simulink model "experiment_setup_R2019b"  (R2020a)
settings: Solver=FixedStepAuto  StartTime=0.0  StopTime=inf  FixedStep=1  RelTol=1e-3
libraries: modbusMatLib x8, simulink x4, realtime_pacer_lib x2
settings Model: Creator=pppc  LastModifiedBy=Casper and Adis
settings DebuggingCC: InheritedTsInSrcMsg=none
settings SFSimCC: CustomCodeUndefinedFunction=UseInterfaceOnly

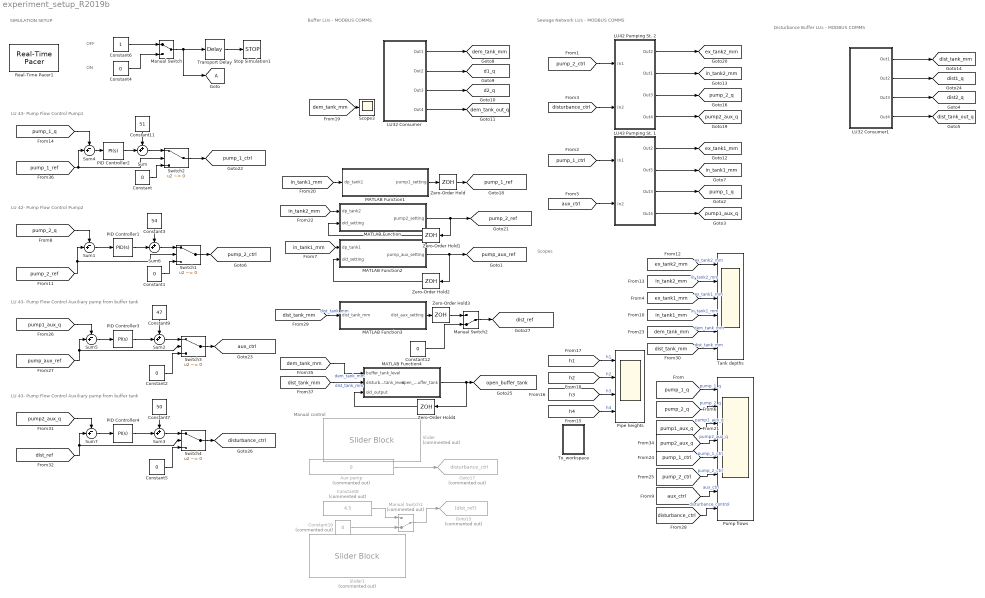
== system experiment_setup_R2019b ==
  note: Buffer LUs - MODBUS COMMS
  note: LU 43- Pump Flow Control Auxiliary pump from buffer tank
  note: Manual control
  note: OFF
  note: SIMULATION SETUP
  note: Sewage Network LUs - MODBUS COMMS
  note: LU 43- Pump Flow Control Pump1
  note: LU 42- Pump Flow Control Pump2
  note: ON
  note: Scopes
  note: Disturbance Buffer LUs - MODBUS COMMS
  note: LU 43- Pump Flow Control Auxiliary pump from buffer tank
  Aux pump : Constant  Commented=on  Value=0
  Constant{,1..2,4..5,12} (6 alike) : Constant  Value=0
  Constant10 : Constant  Commented=on  Value=0
  Constant11 : Constant  Value=51
  Constant3 : Constant  Value=54
  Constant6 : Constant
  Constant7 : Constant  Value=50
  Constant8 : Constant  Commented=on  Value=4.5
  Constant9 : Constant  Value=47
  Goto15 : Goto  Commented=on  GotoTag=dist_ref
  Goto17 : Goto  Commented=on  GotoTag=disturbance_ctrl  TagVisibility=global
  LU32 Consumer : Subsystem
  LU32 Consumer1 : Subsystem
  LU42 Pumping St. 2 : Subsystem
  LU43 Pumping St. 1 : Subsystem
  MATLAB Function : MATLAB Function  TreatAsAtomicUnit=on
  MATLAB Function1 : MATLAB Function  TreatAsAtomicUnit=on
  MATLAB Function2 : MATLAB Function  TreatAsAtomicUnit=on
  MATLAB Function3 : MATLAB Function  TreatAsAtomicUnit=on
  MATLAB Function4 : MATLAB Function  TreatAsAtomicUnit=on
  Manual Switch : ManualSwitch
  Manual Switch1 : ManualSwitch  Commented=on  CurrentSetting=0
  Manual Switch2 : ManualSwitch  CurrentSetting=0
  PID Controller1 : simulink/Continuous/PID Controller  Controller=PID  Form=Parallel  TimeDomain=Continuous-time  UseExternalTs=off  SampleTime=1  IntegratorMethod=Forward Euler  FilterMethod=Forward Euler  ControllerParametersSource=internal  P=0.145  I=0.61  D=0  UseFilter=on  N=100  TunerSelectOption=Transfer Function Based (PID Tuner App)  InitialConditionSource=internal  InitialConditionForIntegrator=0  InitialConditionForFilter=0  DifferentiatorICPrevScaledInput=0  ExternalReset=none  TrackingMode=off  Kt=1  LimitOutput=on  UpperSaturationLimit=46  LowerSaturationLimit=0  LinearizeAsGain=off  AntiWindupMode=clamping  Kb=1  POutMin=[]  POutMax=[]  IOutMin=[]  IOutMax=[]  DOutMin=[]  DOutMax=[]  NOutMin=[]  NOutMax=[]  SumOutMin=[]  SumOutMax=[]  SaturationOutMin=[]  SaturationOutMax=[]  PParamMin=[]  PParamMax=[]  IParamMin=[]  IParamMax=[]  DParamMin=[]  DParamMax=[]  NParamMin=[]  NParamMax=[]  KbParamMin=[]  KbParamMax=[]  KtParamMin=[]  KtParamMax=[]  KbOutMin=[]  KbOutMax=[]  KtOutMin=[]  KtOutMax=[]  IntegratorOutMin=[]  IntegratorOutMax=[]  FilterOutMin=[]  FilterOutMax=[]  SumI1OutMin=[]  SumI1OutMax=[]  SumI2OutMin=[]  SumI2OutMax=[]  SumI3OutMin=[]  SumI3OutMax=[]  SumI4OutMin=[]  SumI4OutMax=[]  SumDOutMin=[]  SumDOutMax=[]  DifferentiatorOutMin=[]  DifferentiatorOutMax=[]  FilterDiffOutCoefMin=[]  FilterDiffOutCoefMax=[]  ReciprocalOutMin=[]  ReciprocalOutMax=[]  SumDenOutMin=[]  SumDenOutMax=[]  SumNumOutMin=[]  SumNumOutMax=[]  DivideOutMin=[]  DivideOutMax=[]  UdiffTsProdOutMin=[]  UdiffTsProdOutMax=[]  NTsProdOutMin=[]  NTsProdOutMax=[]  UintegralTsProdOutMin=[]  UintegralTsProdOutMax=[]  UngainTsProdOutMin=[]  UngainTsProdOutMax=[]  IntegratorContinuousStateAttributes=''  IntegratorStateMustResolveToSignalObject=off  IntegratorRTWStateStorageClass=Auto  FilterContinuousStateAttributes=''  FilterStateMustResolveToSignalObject=off  FilterRTWStateStorageClass=Auto  ParallelPVariant=InternalParameters  IdealPVariant=Disabled  IVariant=InternalParameters  DVariant=InternalParameters  IntegratorVariant=Continuous  SatVariant=Enabled  AWVariant=ContClampingParallel  PCopyVariant=Disabled  TRVariant=Disabled  FdbkBlocksVariant=Forward  IdealPFdbkVariant=Disabled  SatFdbkVariant=Disabled  DerivativeFilterVariant=ContFilter  NVariant=InternalParameters  NCopyVariant=Disabled  FilterICVariant=InternalICsFilter  IntegratorICVariant=InternalICs  ExternalResetVariant=Disabled  TRSumVariant=Passthrough  SumFdbkVariant=Disabled  SumVariant=Sum_PID  TsampFilterVariant=InternalTs  TsampNgainVariant=Passthrough  TsampIntegralVariant=Passthrough
  PID Controller2 : simulink/Continuous/PID Controller  Controller=PI  Form=Parallel  TimeDomain=Continuous-time  UseExternalTs=off  SampleTime=1  IntegratorMethod=Forward Euler  FilterMethod=Forward Euler  ControllerParametersSource=internal  P=0.1  I=0.3  D=0  UseFilter=on  N=100  TunerSelectOption=Transfer Function Based (PID Tuner App)  InitialConditionSource=internal  InitialConditionForIntegrator=0  InitialConditionForFilter=0  DifferentiatorICPrevScaledInput=0  ExternalReset=none  TrackingMode=off  Kt=1  LimitOutput=on  UpperSaturationLimit=49  LowerSaturationLimit=0  LinearizeAsGain=off  AntiWindupMode=clamping  Kb=1  POutMin=[]  POutMax=[]  IOutMin=[]  IOutMax=[]  DOutMin=[]  DOutMax=[]  NOutMin=[]  NOutMax=[]  SumOutMin=[]  SumOutMax=[]  SaturationOutMin=[]  SaturationOutMax=[]  PParamMin=[]  PParamMax=[]  IParamMin=[]  IParamMax=[]  DParamMin=[]  DParamMax=[]  NParamMin=[]  NParamMax=[]  KbParamMin=[]  KbParamMax=[]  KtParamMin=[]  KtParamMax=[]  KbOutMin=[]  KbOutMax=[]  KtOutMin=[]  KtOutMax=[]  IntegratorOutMin=[]  IntegratorOutMax=[]  FilterOutMin=[]  FilterOutMax=[]  SumI1OutMin=[]  SumI1OutMax=[]  SumI2OutMin=[]  SumI2OutMax=[]  SumI3OutMin=[]  SumI3OutMax=[]  SumI4OutMin=[]  SumI4OutMax=[]  SumDOutMin=[]  SumDOutMax=[]  DifferentiatorOutMin=[]  DifferentiatorOutMax=[]  FilterDiffOutCoefMin=[]  FilterDiffOutCoefMax=[]  ReciprocalOutMin=[]  ReciprocalOutMax=[]  SumDenOutMin=[]  SumDenOutMax=[]  SumNumOutMin=[]  SumNumOutMax=[]  DivideOutMin=[]  DivideOutMax=[]  UdiffTsProdOutMin=[]  UdiffTsProdOutMax=[]  NTsProdOutMin=[]  NTsProdOutMax=[]  UintegralTsProdOutMin=[]  UintegralTsProdOutMax=[]  UngainTsProdOutMin=[]  UngainTsProdOutMax=[]  IntegratorContinuousStateAttributes=''  IntegratorStateMustResolveToSignalObject=off  IntegratorRTWStateStorageClass=Auto  FilterContinuousStateAttributes=''  FilterStateMustResolveToSignalObject=off  FilterRTWStateStorageClass=Auto  ParallelPVariant=InternalParameters  IdealPVariant=Disabled  IVariant=InternalParameters  DVariant=Disabled  IntegratorVariant=Continuous  SatVariant=Enabled  AWVariant=ContClampingParallel  PCopyVariant=Disabled  TRVariant=Disabled  FdbkBlocksVariant=Forward  IdealPFdbkVariant=Disabled  SatFdbkVariant=Disabled  DerivativeFilterVariant=Disabled  NVariant=Disabled  NCopyVariant=Disabled_SignalSpec  FilterICVariant=Disabled  IntegratorICVariant=InternalICs  ExternalResetVariant=Disabled  TRSumVariant=Passthrough  SumFdbkVariant=Disabled  SumVariant=Sum_PI  TsampFilterVariant=InternalTs  TsampNgainVariant=Passthrough  TsampIntegralVariant=Passthrough
  PID Controller3 : simulink/Continuous/PID Controller  Controller=PI  Form=Parallel  TimeDomain=Continuous-time  UseExternalTs=off  SampleTime=1  IntegratorMethod=Forward Euler  FilterMethod=Forward Euler  ControllerParametersSource=internal  P=0.15  I=0.45  D=0  UseFilter=on  N=100  TunerSelectOption=Transfer Function Based (PID Tuner App)  InitialConditionSource=internal  InitialConditionForIntegrator=0  InitialConditionForFilter=0  DifferentiatorICPrevScaledInput=0  ExternalReset=none  TrackingMode=off  Kt=1  LimitOutput=on  UpperSaturationLimit=53  LowerSaturationLimit=0  LinearizeAsGain=off  AntiWindupMode=clamping  Kb=1  POutMin=[]  POutMax=[]  IOutMin=[]  IOutMax=[]  DOutMin=[]  DOutMax=[]  NOutMin=[]  NOutMax=[]  SumOutMin=[]  SumOutMax=[]  SaturationOutMin=[]  SaturationOutMax=[]  PParamMin=[]  PParamMax=[]  IParamMin=[]  IParamMax=[]  DParamMin=[]  DParamMax=[]  NParamMin=[]  NParamMax=[]  KbParamMin=[]  KbParamMax=[]  KtParamMin=[]  KtParamMax=[]  KbOutMin=[]  KbOutMax=[]  KtOutMin=[]  KtOutMax=[]  IntegratorOutMin=[]  IntegratorOutMax=[]  FilterOutMin=[]  FilterOutMax=[]  SumI1OutMin=[]  SumI1OutMax=[]  SumI2OutMin=[]  SumI2OutMax=[]  SumI3OutMin=[]  SumI3OutMax=[]  SumI4OutMin=[]  SumI4OutMax=[]  SumDOutMin=[]  SumDOutMax=[]  DifferentiatorOutMin=[]  DifferentiatorOutMax=[]  FilterDiffOutCoefMin=[]  FilterDiffOutCoefMax=[]  ReciprocalOutMin=[]  ReciprocalOutMax=[]  SumDenOutMin=[]  SumDenOutMax=[]  SumNumOutMin=[]  SumNumOutMax=[]  DivideOutMin=[]  DivideOutMax=[]  UdiffTsProdOutMin=[]  UdiffTsProdOutMax=[]  NTsProdOutMin=[]  NTsProdOutMax=[]  UintegralTsProdOutMin=[]  UintegralTsProdOutMax=[]  UngainTsProdOutMin=[]  UngainTsProdOutMax=[]  IntegratorContinuousStateAttributes=''  IntegratorStateMustResolveToSignalObject=off  IntegratorRTWStateStorageClass=Auto  FilterContinuousStateAttributes=''  FilterStateMustResolveToSignalObject=off  FilterRTWStateStorageClass=Auto  ParallelPVariant=InternalParameters  IdealPVariant=Disabled  IVariant=InternalParameters  DVariant=Disabled  IntegratorVariant=Continuous  SatVariant=Enabled  AWVariant=ContClampingParallel  PCopyVariant=Disabled  TRVariant=Disabled  FdbkBlocksVariant=Forward  IdealPFdbkVariant=Disabled  SatFdbkVariant=Disabled  DerivativeFilterVariant=Disabled  NVariant=Disabled  NCopyVariant=Disabled_SignalSpec  FilterICVariant=Disabled  IntegratorICVariant=InternalICs  ExternalResetVariant=Disabled  TRSumVariant=Passthrough  SumFdbkVariant=Disabled  SumVariant=Sum_PI  TsampFilterVariant=InternalTs  TsampNgainVariant=Passthrough  TsampIntegralVariant=Passthrough
  PID Controller4 : simulink/Continuous/PID Controller  Controller=PI  Form=Parallel  TimeDomain=Continuous-time  UseExternalTs=off  SampleTime=1  IntegratorMethod=Forward Euler  FilterMethod=Forward Euler  ControllerParametersSource=internal  P=0.1  I=0.4  D=0  UseFilter=on  N=100  TunerSelectOption=Transfer Function Based (PID Tuner App)  InitialConditionSource=internal  InitialConditionForIntegrator=0  InitialConditionForFilter=0  DifferentiatorICPrevScaledInput=0  ExternalReset=none  TrackingMode=off  Kt=1  LimitOutput=on  UpperSaturationLimit=53  LowerSaturationLimit=0  LinearizeAsGain=off  AntiWindupMode=clamping  Kb=1  POutMin=[]  POutMax=[]  IOutMin=[]  IOutMax=[]  DOutMin=[]  DOutMax=[]  NOutMin=[]  NOutMax=[]  SumOutMin=[]  SumOutMax=[]  SaturationOutMin=[]  SaturationOutMax=[]  PParamMin=[]  PParamMax=[]  IParamMin=[]  IParamMax=[]  DParamMin=[]  DParamMax=[]  NParamMin=[]  NParamMax=[]  KbParamMin=[]  KbParamMax=[]  KtParamMin=[]  KtParamMax=[]  KbOutMin=[]  KbOutMax=[]  KtOutMin=[]  KtOutMax=[]  IntegratorOutMin=[]  IntegratorOutMax=[]  FilterOutMin=[]  FilterOutMax=[]  SumI1OutMin=[]  SumI1OutMax=[]  SumI2OutMin=[]  SumI2OutMax=[]  SumI3OutMin=[]  SumI3OutMax=[]  SumI4OutMin=[]  SumI4OutMax=[]  SumDOutMin=[]  SumDOutMax=[]  DifferentiatorOutMin=[]  DifferentiatorOutMax=[]  FilterDiffOutCoefMin=[]  FilterDiffOutCoefMax=[]  ReciprocalOutMin=[]  ReciprocalOutMax=[]  SumDenOutMin=[]  SumDenOutMax=[]  SumNumOutMin=[]  SumNumOutMax=[]  DivideOutMin=[]  DivideOutMax=[]  UdiffTsProdOutMin=[]  UdiffTsProdOutMax=[]  NTsProdOutMin=[]  NTsProdOutMax=[]  UintegralTsProdOutMin=[]  UintegralTsProdOutMax=[]  UngainTsProdOutMin=[]  UngainTsProdOutMax=[]  IntegratorContinuousStateAttributes=''  IntegratorStateMustResolveToSignalObject=off  IntegratorRTWStateStorageClass=Auto  FilterContinuousStateAttributes=''  FilterStateMustResolveToSignalObject=off  FilterRTWStateStorageClass=Auto  ParallelPVariant=InternalParameters  IdealPVariant=Disabled  IVariant=InternalParameters  DVariant=Disabled  IntegratorVariant=Continuous  SatVariant=Enabled  AWVariant=ContClampingParallel  PCopyVariant=Disabled  TRVariant=Disabled  FdbkBlocksVariant=Forward  IdealPFdbkVariant=Disabled  SatFdbkVariant=Disabled  DerivativeFilterVariant=Disabled  NVariant=Disabled  NCopyVariant=Disabled_SignalSpec  FilterICVariant=Disabled  IntegratorICVariant=InternalICs  ExternalResetVariant=Disabled  TRSumVariant=Passthrough  SumFdbkVariant=Disabled  SumVariant=Sum_PI  TsampFilterVariant=InternalTs  TsampNgainVariant=Passthrough  TsampIntegralVariant=Passthrough
  Pipe heights : Scope  NumInputPorts=4
  Pump flows : Scope  NumInputPorts=8
  Real-Time Pacer1 : realtime_pacer_lib/Real-Time Pacer  simTimePerRealTime=2
  Scope3 : Scope
  Slider : SliderBlock  Commented=on
  Slider1 : SliderBlock  Commented=on  ScaleMax=9.5
  Stop Simulation1 : Stop
  Sum{,2..3,6} (4 alike) : Sum  Inputs=++|
  Sum{1,4..5,7} (4 alike) : Sum  Inputs=-+|
  Switch{1..4} (4 alike) : Switch  Criteria=u2 ~= 0
  Tank depths : Scope  NumInputPorts=6
  To_workspace : Subsystem
  Transport Delay : TransportDelay  DelayTime=2
  Zero-Order Hold : ZeroOrderHold  SampleTime=60
  Zero-Order Hold1 : ZeroOrderHold  SampleTime=2
  Zero-Order Hold2 : ZeroOrderHold  SampleTime=2
  Zero-Order Hold3 : ZeroOrderHold  SampleTime=30
  Zero-Order Hold4 : ZeroOrderHold  SampleTime=2
  tag scope: A=global, aux_ctrl=global, d1_q=global, d2_q=global, dem_tank_mm=global, dem_tank_out_q=global, dist1_q=global, dist2_q=global, dist_ref=global, dist_tank_mm=global, dist_tank_out_q=global, disturbance_ctrl=global, ex_tank1_mm=global, ex_tank2_mm=global, in_tank1_mm=global, in_tank2_mm=global, open_buffer_tank=global, pump1_aux_q=global, pump2_aux_q=global, pump_1_ctrl=global, pump_1_q=global, pump_1_ref=global, pump_2_ctrl=global, pump_2_q=global, pump_2_ref=global, pump_aux_ref=global
  wires:
  [pump_1_q] -> Sum4/1
  [pump_aux_ref] -> Sum5/2, Switch3/2
  [disturbance_ctrl] -> LU42 Pumping St. 2/2(In2)
  [pump_2_ref] -> Switch1/2, Sum1/2
  [in_tank2_mm] -> Tank depths/2  "in_tank2_mm"
  [dem_tank_mm] -> Scope3/1
  MATLAB Function/1(pump2_setting) -> Zero-Order Hold1/1, [pump_2_ref]
  [pump_2_q] -> Pump flows/2  "pump_2_q"
  Switch1/1 -> [pump_2_ctrl]
  Sum6/1 -> Switch1/1
  PID Controller2/1 -> Sum/2
  PID Controller1/1 -> Sum6/2
  Switch3/1 -> [aux_ctrl]
  [pump_2_q] -> Sum1/1
  Sum2/1 -> Switch3/1
  LU42 Pumping St. 2/3(Out3) -> [pump_2_q]
  Zero-Order Hold/1 -> [pump_1_ref]
  Constant9/1 -> Sum2/1
  LU32 Consumer/4(Out4) -> [dem_tank_out_q]
  Constant2/1 -> Switch3/3
  PID Controller3/1 -> Sum2/2
  [h4] -> Pipe heights/4  "h4"
  Constant11/1 -> Sum/1
  [pump_1_ref] -> Sum4/2, Switch2/2
  [pump_1_ctrl] -> LU43 Pumping St. 1/1(In1)
  Constant3/1 -> Sum6/1
  LU43 Pumping St. 1/2(Out5) -> [in_tank1_mm]
  Sum/1 -> Switch2/1
  Transport Delay/1 -> Stop Simulation1/1
  Constant6/1 -> Manual Switch/1
  Constant/1 -> Switch2/3
  LU43 Pumping St. 1/1(Out2) -> [ex_tank1_mm]
  [in_tank1_mm] -> Tank depths/4  "in_tank1_mm"
  Aux pump/1 -> Goto17/1
  Constant4/1 -> Manual Switch/2
  [ex_tank1_mm] -> Tank depths/3  "ex_tank1_mm"
  [pump1_aux_q] -> Sum5/1
  [dem_tank_mm] -> Tank depths/5  "dem_tank_mm"
  Sum5/1 -> PID Controller3/1
  Manual Switch/1 -> [A], Transport Delay/1
  [pump_2_ctrl] -> LU42 Pumping St. 2/1(In1)
  LU42 Pumping St. 2/4(Out4) -> [pump2_aux_q]
  LU32 Consumer/3(Out3) -> [d2_q]
  LU32 Consumer/1(Out1) -> [dem_tank_mm]
  LU42 Pumping St. 2/1(Out2) -> [ex_tank2_mm]
  [in_tank1_mm] -> MATLAB Function1/1(dp_tank1)
  [in_tank2_mm] -> MATLAB Function/1(dp_tank2)
  Sum1/1 -> PID Controller1/1
  [ex_tank2_mm] -> Tank depths/1  "ex_tank2_mm"
  Switch2/1 -> [pump_1_ctrl]
  [h2] -> Pipe heights/2  "h2"
  [h3] -> Pipe heights/3  "h3"
  LU43 Pumping St. 1/3(Out3) -> [pump_1_q]
  Sum4/1 -> PID Controller2/1
  LU43 Pumping St. 1/4(Out4) -> [pump1_aux_q]
  [aux_ctrl] -> LU43 Pumping St. 1/2(In2)
  LU42 Pumping St. 2/2(Out1) -> [in_tank2_mm]
  LU32 Consumer/2(Out2) -> [d1_q]
  MATLAB Function1/1(pump1_setting) -> Zero-Order Hold/1
  Constant1/1 -> Switch1/3
  [in_tank1_mm] -> MATLAB Function2/1(dp_tank1)
  MATLAB Function2/1(pump_aux_setting) -> Zero-Order Hold2/1, [pump_aux_ref]
  Zero-Order Hold1/1 -> MATLAB Function/2(old_setting)
  Zero-Order Hold2/1 -> MATLAB Function2/2(old_setting)
  [pump1_aux_q] -> Pump flows/3  "pump1_aux_q"
  [pump_1_q] -> Pump flows/1  "pump_1_q"
  LU32 Consumer1/2(Out2) -> [dist1_q]
  LU32 Consumer1/3(Out3) -> [dist2_q]
  LU32 Consumer1/4(Out4) -> [dist_tank_out_q]
  LU32 Consumer1/1(Out1) -> [dist_tank_mm]
  [dist_tank_mm] -> Tank depths/6  "dist_tank_mm"
  [pump2_aux_q] -> Sum7/1
  Constant7/1 -> Sum3/1
  Switch4/1 -> [disturbance_ctrl]
  PID Controller4/1 -> Sum3/2
  [dist_ref] -> Sum7/2, Switch4/2
  Sum3/1 -> Switch4/1
  Sum7/1 -> PID Controller4/1
  Constant5/1 -> Switch4/3
  [pump_1_ctrl] -> Pump flows/5  "pump_1_ctrl"
  [pump_2_ctrl] -> Pump flows/6  "pump_2_ctrl"
  [aux_ctrl] -> Pump flows/7  "aux_ctrl"
  [disturbance_ctrl] -> Pump flows/8  "disturbance_control"
  [pump2_aux_q] -> Pump flows/4  "pump2_aux_q"
  [dem_tank_mm] -> MATLAB Function4/1(buffer_tank_level)  "dem_tank_mm"
  [dist_tank_mm] -> MATLAB Function4/2(disturbance_tank_level)  "dist_tank_mm"
  MATLAB Function4/1(open_buffer_tank) -> Zero-Order Hold4/1, [open_buffer_tank]
  Zero-Order Hold4/1 -> MATLAB Function4/3(old_output)
  [h1] -> Pipe heights/1  "h1"
  Constant8/1 -> Manual Switch1/1
  Constant10/1 -> Manual Switch1/2
  Manual Switch1/1 -> Goto15/1
  [dist_tank_mm] -> MATLAB Function3/1(dist_tank_mm)  "dist_tank_mm"
  MATLAB Function3/1(dist_aux_setting) -> Zero-Order Hold3/1
  Zero-Order Hold3/1 -> Manual Switch2/1
  Manual Switch2/1 -> [dist_ref]
  Constant12/1 -> Manual Switch2/2

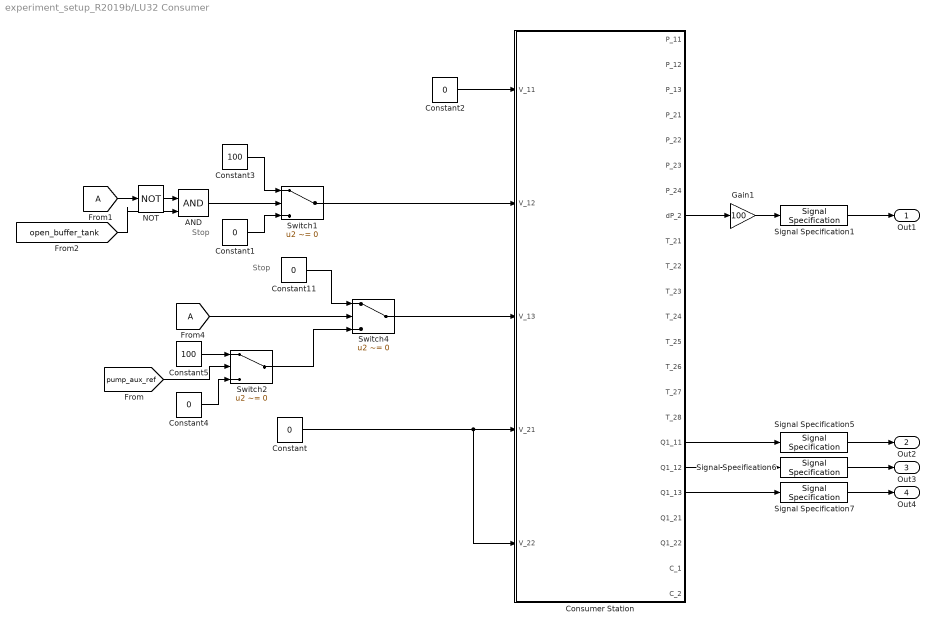
== system experiment_setup_R2019b/LU32 Consumer ==
  note: Stop
  note: Stop
  AND : Logic  IconShape=distinctive  AllPortsSameDT=off  OutDataTypeStr=boolean
  Constant{,1..2,4,11} (5 alike) : Constant  Value=0
  Constant3 : Constant  Value=100
  Constant5 : Constant  Value=100
  Consumer Station : Subsystem
  Gain1 : Gain  Gain=100
  NOT : Logic  Operator=NOT  IconShape=distinctive  AllPortsSameDT=off  OutDataTypeStr=boolean
  Signal Specification1 : SignalSpecification  Unit=mm
  Signal Specification5 : SignalSpecification  Unit=l/min
  Signal Specification6 : SignalSpecification  Unit=l/min
  Signal Specification7 : SignalSpecification  Unit=l/min
  Switch1 : Switch  Criteria=u2 ~= 0
  Switch2 : Switch  Criteria=u2 ~= 0
  Switch4 : Switch  Criteria=u2 ~= 0
  Out1 : Outport  VectorParamsAs1DForOutWhenUnconnected=off
  Out2 : Outport  Port=2  VectorParamsAs1DForOutWhenUnconnected=off
  Out3 : Outport  Port=3  VectorParamsAs1DForOutWhenUnconnected=off
  Out4 : Outport  Port=4  VectorParamsAs1DForOutWhenUnconnected=off
  wires:
  Consumer Station/8(dP_2) -> Gain1/1
  Switch4/1 -> Consumer Station/3(V_13)
  Consumer Station/19(Q1_13) -> Signal Specification7/1
  Consumer Station/17(Q1_11) -> Signal Specification5/1
  Consumer Station/18(Q1_12) -> Signal Specification6/1
  Gain1/1 -> Signal Specification1/1
  [A] -> Switch4/2
  Signal Specification7/1 -> Out4/1
  Constant11/1 -> Switch4/1
  Signal Specification5/1 -> Out2/1
  Constant/1 -> Consumer Station/5(V_22), Consumer Station/4(V_21)
  Signal Specification6/1 -> Out3/1
  Signal Specification1/1 -> Out1/1
  Switch1/1 -> Consumer Station/2(V_12)
  Constant2/1 -> Consumer Station/1(V_11)
  [pump_aux_ref] -> Switch2/2
  Switch2/1 -> Switch4/3
  Constant5/1 -> Switch2/1
  Constant4/1 -> Switch2/3
  [A] -> NOT/1
  NOT/1 -> AND/1
  AND/1 -> Switch1/2
  Constant1/1 -> Switch1/3
  Constant3/1 -> Switch1/1
  [open_buffer_tank] -> AND/2

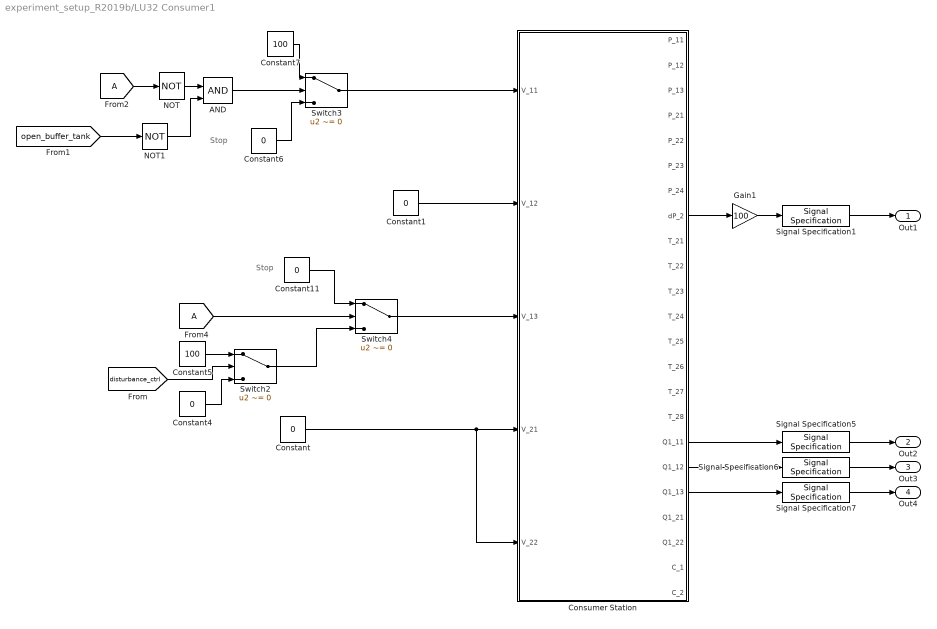
== system experiment_setup_R2019b/LU32 Consumer1 ==
  note: Stop
  note: Stop
  AND : Logic  IconShape=distinctive  AllPortsSameDT=off  OutDataTypeStr=boolean
  Constant{,1,4,6,11} (5 alike) : Constant  Value=0
  Constant5 : Constant  Value=100
  Constant7 : Constant  Value=100
  Consumer Station : Subsystem
  Gain1 : Gain  Gain=100
  NOT : Logic  Operator=NOT  IconShape=distinctive  AllPortsSameDT=off  OutDataTypeStr=boolean
  NOT1 : Logic  Operator=NOT  IconShape=distinctive  AllPortsSameDT=off  OutDataTypeStr=boolean
  Signal Specification1 : SignalSpecification  Unit=mm
  Signal Specification5 : SignalSpecification  Unit=l/min
  Signal Specification6 : SignalSpecification  Unit=l/min
  Signal Specification7 : SignalSpecification  Unit=l/min
  Switch2 : Switch  Criteria=u2 ~= 0
  Switch3 : Switch  Criteria=u2 ~= 0
  Switch4 : Switch  Criteria=u2 ~= 0
  Out1 : Outport  VectorParamsAs1DForOutWhenUnconnected=off
  Out2 : Outport  Port=2  VectorParamsAs1DForOutWhenUnconnected=off
  Out3 : Outport  Port=3  VectorParamsAs1DForOutWhenUnconnected=off
  Out4 : Outport  Port=4  VectorParamsAs1DForOutWhenUnconnected=off
  wires:
  Consumer Station/8(dP_2) -> Gain1/1
  Switch4/1 -> Consumer Station/3(V_13)
  Consumer Station/19(Q1_13) -> Signal Specification7/1
  Consumer Station/17(Q1_11) -> Signal Specification5/1
  Consumer Station/18(Q1_12) -> Signal Specification6/1
  Gain1/1 -> Signal Specification1/1
  [A] -> Switch4/2
  Signal Specification7/1 -> Out4/1
  Constant11/1 -> Switch4/1
  Signal Specification5/1 -> Out2/1
  Constant/1 -> Consumer Station/5(V_22), Consumer Station/4(V_21)
  Signal Specification6/1 -> Out3/1
  Signal Specification1/1 -> Out1/1
  Switch3/1 -> Consumer Station/1(V_11)
  [disturbance_ctrl] -> Switch2/2
  Switch2/1 -> Switch4/3
  Constant5/1 -> Switch2/1
  Constant4/1 -> Switch2/3
  Constant1/1 -> Consumer Station/2(V_12)
  [A] -> NOT/1
  Constant6/1 -> Switch3/3
  Constant7/1 -> Switch3/1
  AND/1 -> Switch3/2
  NOT/1 -> AND/1
  [open_buffer_tank] -> NOT1/1
  NOT1/1 -> AND/2

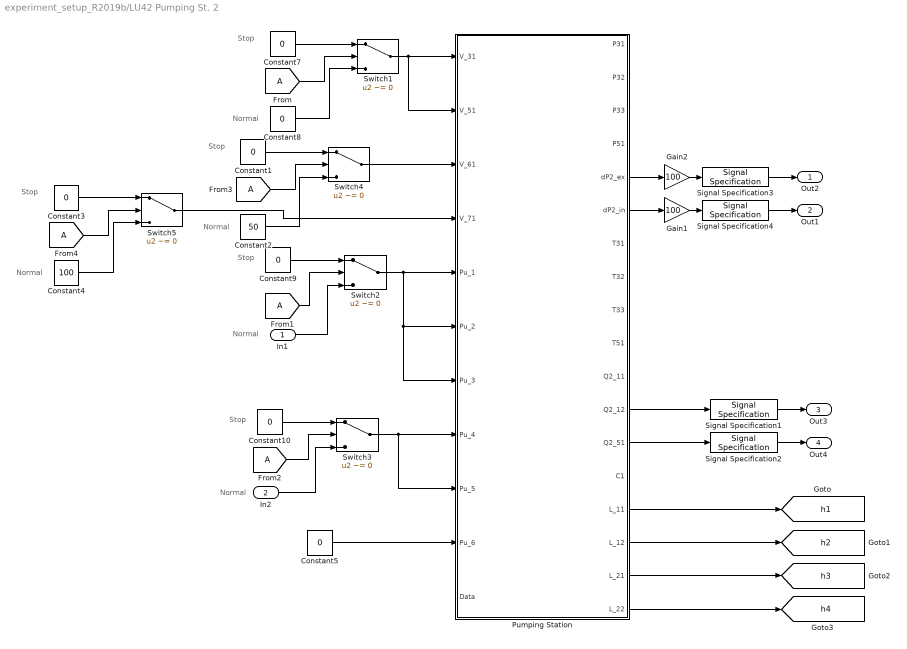
== system experiment_setup_R2019b/LU42 Pumping St. 2 ==
  note: Stop
  note: Stop
  note: Normal
  note: Stop
  note: Normal
  note: Normal
  note: Stop
  note: Normal
  note: Normal
  note: Stop
  In1 : Inport
  In2 : Inport  Port=2
  Constant{1,3,5,7..10} (7 alike) : Constant  Value=0
  Constant2 : Constant  Value=50
  Constant4 : Constant  Value=100
  Gain1 : Gain  Gain=100
  Gain2 : Gain  Gain=100
  Pumping Station : Subsystem
  Signal Specification1 : SignalSpecification  Unit=l/min
  Signal Specification2 : SignalSpecification  Unit=l/min
  Signal Specification3 : SignalSpecification  Unit=mm
  Signal Specification4 : SignalSpecification  Unit=mm
  Switch{1..5} (5 alike) : Switch  Criteria=u2 ~= 0
  Out2 : Outport  VectorParamsAs1DForOutWhenUnconnected=off
  Out1 : Outport  Port=2  VectorParamsAs1DForOutWhenUnconnected=off
  Out3 : Outport  Port=3  VectorParamsAs1DForOutWhenUnconnected=off
  Out4 : Outport  Port=4  VectorParamsAs1DForOutWhenUnconnected=off
  tag scope: h1=global, h2=global, h3=global, h4=global
  wires:
  Switch2/1 -> Pumping Station/7(Pu_3), Pumping Station/6(Pu_2), Pumping Station/5(Pu_1)
  [A] -> Switch1/2
  Constant7/1 -> Switch1/1
  Constant8/1 -> Switch1/3
  Switch3/1 -> Pumping Station/9(Pu_5), Pumping Station/8(Pu_4)
  Constant10/1 -> Switch3/1
  In1/1 -> Switch2/3
  [A] -> Switch2/2
  Constant9/1 -> Switch2/1
  In2/1 -> Switch3/3
  Gain2/1 -> Signal Specification3/1
  Constant5/1 -> Pumping Station/10(Pu_6)
  Signal Specification3/1 -> Out2/1
  [A] -> Switch3/2
  Pumping Station/5(dP2_ex) -> Gain2/1
  Switch1/1 -> Pumping Station/2(V_51), Pumping Station/1(V_31)
  Signal Specification1/1 -> Out3/1
  Signal Specification2/1 -> Out4/1
  Pumping Station/12(Q2_12) -> Signal Specification1/1
  Pumping Station/13(Q2_51) -> Signal Specification2/1
  Pumping Station/6(dP2_in) -> Gain1/1
  Gain1/1 -> Signal Specification4/1
  Signal Specification4/1 -> Out1/1
  Pumping Station/15(L_11) -> [h1]
  Pumping Station/17(L_21) -> [h3]
  Pumping Station/18(L_22) -> [h4]
  Constant1/1 -> Switch4/1
  Constant2/1 -> Switch4/3
  [A] -> Switch4/2
  Switch4/1 -> Pumping Station/3(V_61)
  Pumping Station/16(L_12) -> [h2]
  Constant4/1 -> Switch5/3
  Constant3/1 -> Switch5/1
  [A] -> Switch5/2
  Switch5/1 -> Pumping Station/4(V_71)

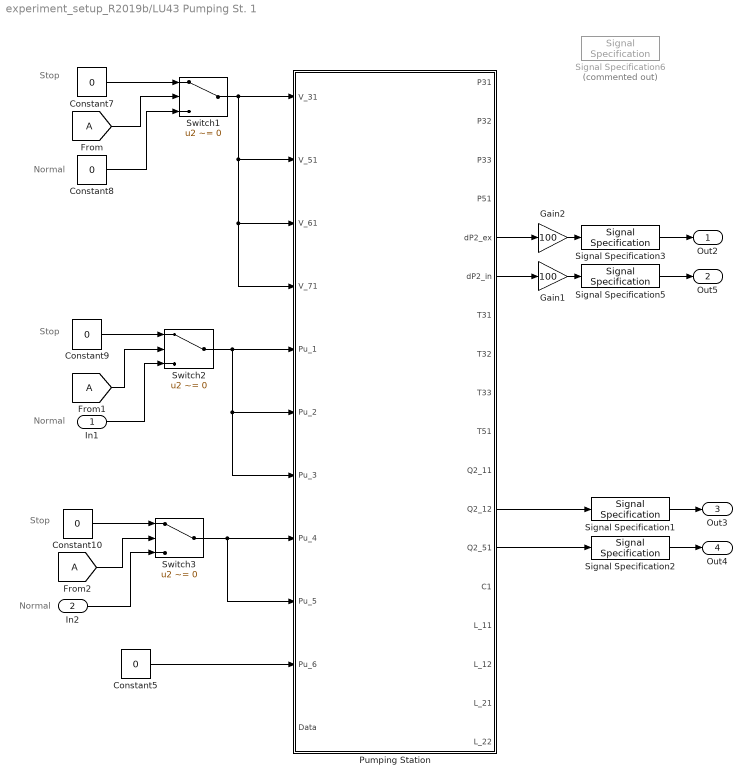
== system experiment_setup_R2019b/LU43 Pumping St. 1 ==
  note: Stop
  note: Stop
  note: Normal
  note: Stop
  note: Normal
  note: Normal
  In1 : Inport
  In2 : Inport  Port=2
  Constant{5,7..10} (5 alike) : Constant  Value=0
  Gain1 : Gain  Gain=100
  Gain2 : Gain  Gain=100
  Pumping Station : Subsystem
  Signal Specification1 : SignalSpecification  Unit=l/min
  Signal Specification2 : SignalSpecification  Unit=l/min
  Signal Specification3 : SignalSpecification  Unit=mm
  Signal Specification5 : SignalSpecification  Unit=mm
  Signal Specification6 : SignalSpecification  Commented=on  Unit=bar
  Switch1 : Switch  Criteria=u2 ~= 0
  Switch2 : Switch  Criteria=u2 ~= 0
  Switch3 : Switch  Criteria=u2 ~= 0
  Out2 : Outport  VectorParamsAs1DForOutWhenUnconnected=off
  Out5 : Outport  Port=2  VectorParamsAs1DForOutWhenUnconnected=off
  Out3 : Outport  Port=3  VectorParamsAs1DForOutWhenUnconnected=off
  Out4 : Outport  Port=4  VectorParamsAs1DForOutWhenUnconnected=off
  wires:
  Switch2/1 -> Pumping Station/7(Pu_3), Pumping Station/6(Pu_2), Pumping Station/5(Pu_1)
  [A] -> Switch1/2
  Constant7/1 -> Switch1/1
  Constant8/1 -> Switch1/3
  Switch3/1 -> Pumping Station/9(Pu_5), Pumping Station/8(Pu_4)
  Constant10/1 -> Switch3/1
  In1/1 -> Switch2/3
  [A] -> Switch2/2
  Constant9/1 -> Switch2/1
  In2/1 -> Switch3/3
  Gain2/1 -> Signal Specification3/1
  Constant5/1 -> Pumping Station/10(Pu_6)
  Signal Specification3/1 -> Out2/1
  [A] -> Switch3/2
  Pumping Station/5(dP2_ex) -> Gain2/1
  Switch1/1 -> Pumping Station/4(V_71), Pumping Station/3(V_61), Pumping Station/2(V_51), Pumping Station/1(V_31)
  Signal Specification1/1 -> Out3/1
  Signal Specification2/1 -> Out4/1
  Pumping Station/12(Q2_12) -> Signal Specification1/1
  Pumping Station/13(Q2_51) -> Signal Specification2/1
  Pumping Station/6(dP2_in) -> Gain1/1
  Signal Specification5/1 -> Out5/1
  Gain1/1 -> Signal Specification5/1

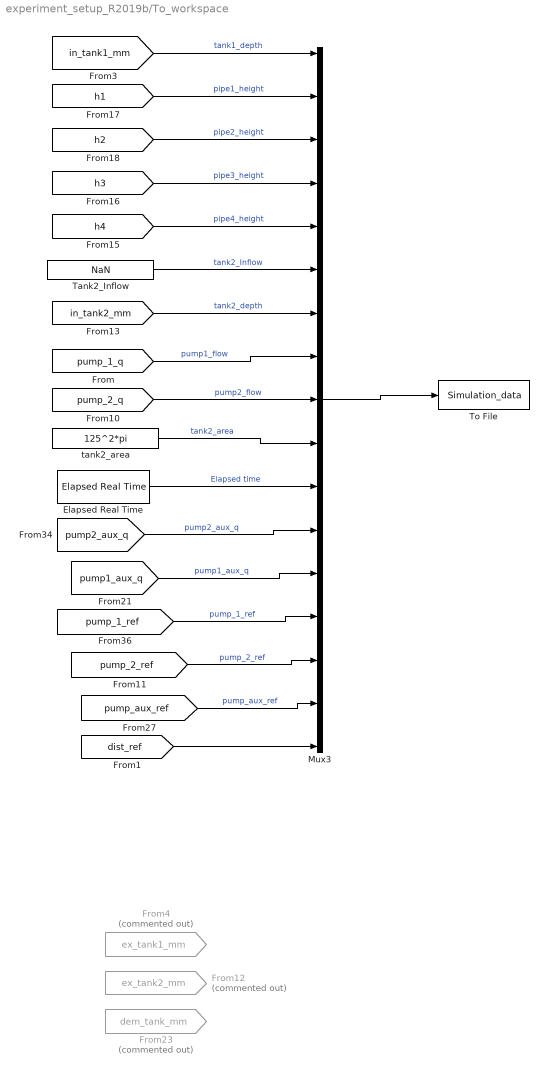
== system experiment_setup_R2019b/To_workspace ==
  Elapsed Real Time : realtime_pacer_lib/Elapsed Real Time
  From12 : From  Commented=on  GotoTag=ex_tank2_mm  TagVisibility=global
  From23 : From  Commented=on  GotoTag=dem_tank_mm  TagVisibility=global
  From4 : From  Commented=on  GotoTag=ex_tank1_mm  TagVisibility=global
  Mux3 : Mux  Inputs=17
  Tank2_Inflow : Constant  Value=NaN
  To File : ToFile  Filename=Simulation_data  SaveFormat=Timeseries
  tank2_area : Constant  Value=125^2*pi
  wires:
  Mux3/1 -> To File/1
  [in_tank1_mm] -> Mux3/1  "tank1_depth"
  [h1] -> Mux3/2  "pipe1_height"
  [h2] -> Mux3/3  "pipe2_height"
  [h3] -> Mux3/4  "pipe3_height"
  [in_tank2_mm] -> Mux3/7  "tank2_depth"
  Tank2_Inflow/1 -> Mux3/6  "tank2_Inflow"
  [h4] -> Mux3/5  "pipe4_height"
  [pump_1_q] -> Mux3/8  "pump1_flow"
  [pump_2_q] -> Mux3/9  "pump2_flow"
  tank2_area/1 -> Mux3/10  "tank2_area"
  Elapsed Real Time/1 -> Mux3/11  "Elapsed time"
  [pump1_aux_q] -> Mux3/13  "pump1_aux_q"
  [pump_1_ref] -> Mux3/14  "pump_1_ref"
  [pump_2_ref] -> Mux3/15  "pump_2_ref"
  [pump_aux_ref] -> Mux3/16  "pump_aux_ref"
  [pump2_aux_q] -> Mux3/12  "pump2_aux_q"
  [dist_ref] -> Mux3/17

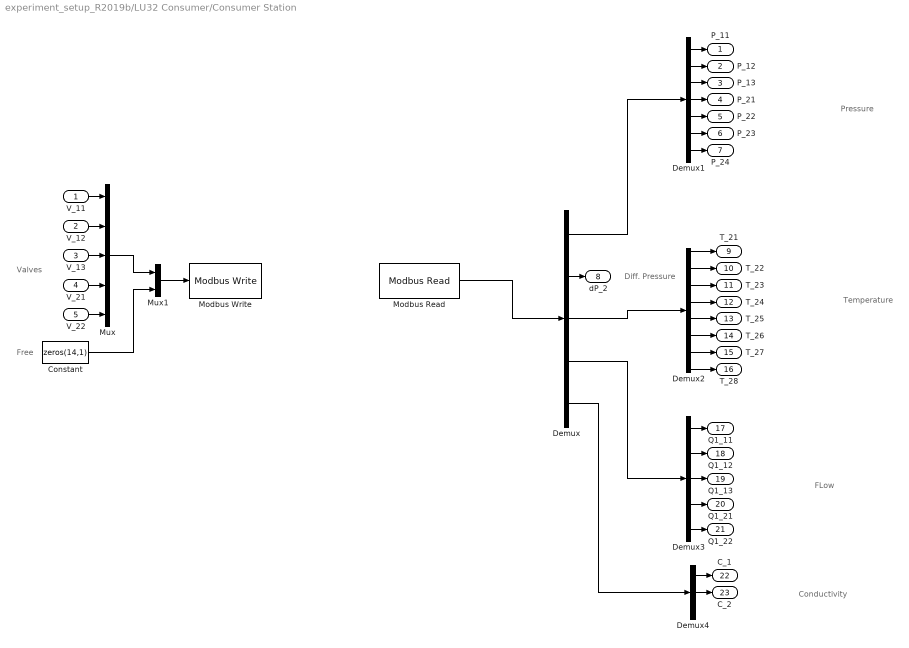
== system experiment_setup_R2019b/LU32 Consumer/Consumer Station ==
  note: Pressure
  note: Temperature
  note: FLow
  note: Conductivity
  note: Valves
  note: Diff. Pressure
  note: Free
  V_11 : Inport
  V_12 : Inport  Port=2
  V_13 : Inport  Port=3
  V_21 : Inport  Port=4
  V_22 : Inport  Port=5
  Constant : Constant  Value=zeros(14,1)
  Demux : Demux  Outputs=[7 1 8 5 3]
  Demux1 : Demux  Outputs=7
  Demux2 : Demux  Outputs=8
  Demux3 : Demux  Outputs=5
  Demux4 : Demux  Outputs=3
  Modbus Read : modbusMatLib/Modbus Read  registry=0  ipAddress='192.168.100.32'  port=502
  Modbus Write : modbusMatLib/Modbus Write  registry=001  port=502  ipAddress='192.168.100.32'
  Mux : Mux  Inputs=5
  Mux1 : Mux  Inputs=2
  P_11 : Outport  VectorParamsAs1DForOutWhenUnconnected=off
  P_12 : Outport  Port=2  VectorParamsAs1DForOutWhenUnconnected=off
  P_13 : Outport  Port=3  VectorParamsAs1DForOutWhenUnconnected=off
  P_21 : Outport  Port=4  VectorParamsAs1DForOutWhenUnconnected=off
  P_22 : Outport  Port=5  VectorParamsAs1DForOutWhenUnconnected=off
  P_23 : Outport  Port=6  VectorParamsAs1DForOutWhenUnconnected=off
  P_24 : Outport  Port=7  VectorParamsAs1DForOutWhenUnconnected=off
  dP_2 : Outport  Port=8  VectorParamsAs1DForOutWhenUnconnected=off
  T_21 : Outport  Port=9  VectorParamsAs1DForOutWhenUnconnected=off
  T_22 : Outport  Port=10  VectorParamsAs1DForOutWhenUnconnected=off
  T_23 : Outport  Port=11  VectorParamsAs1DForOutWhenUnconnected=off
  T_24 : Outport  Port=12  VectorParamsAs1DForOutWhenUnconnected=off
  T_25 : Outport  Port=13  VectorParamsAs1DForOutWhenUnconnected=off
  T_26 : Outport  Port=14  VectorParamsAs1DForOutWhenUnconnected=off
  T_27 : Outport  Port=15  VectorParamsAs1DForOutWhenUnconnected=off
  T_28 : Outport  Port=16  VectorParamsAs1DForOutWhenUnconnected=off
  Q1_11 : Outport  Port=17  VectorParamsAs1DForOutWhenUnconnected=off
  Q1_12 : Outport  Port=18  VectorParamsAs1DForOutWhenUnconnected=off
  Q1_13 : Outport  Port=19  VectorParamsAs1DForOutWhenUnconnected=off
  Q1_21 : Outport  Port=20  VectorParamsAs1DForOutWhenUnconnected=off
  Q1_22 : Outport  Port=21  VectorParamsAs1DForOutWhenUnconnected=off
  C_1 : Outport  Port=22  VectorParamsAs1DForOutWhenUnconnected=off
  C_2 : Outport  Port=23  VectorParamsAs1DForOutWhenUnconnected=off
  wires:
  Mux/1 -> Mux1/1
  Mux1/1 -> Modbus Write/1
  Constant/1 -> Mux1/2
  Demux1/5 -> P_22/1
  V_12/1 -> Mux/2
  Demux1/6 -> P_23/1
  Demux1/3 -> P_13/1
  Demux1/4 -> P_21/1
  V_13/1 -> Mux/3
  Demux3/2 -> Q1_12/1
  Demux3/5 -> Q1_22/1
  Demux/2 -> dP_2/1
  Demux3/1 -> Q1_11/1
  Demux1/2 -> P_12/1
  Demux2/5 -> T_25/1
  Demux4/1 -> C_1/1
  V_21/1 -> Mux/4
  Demux3/3 -> Q1_13/1
  Demux1/1 -> P_11/1
  Demux3/4 -> Q1_21/1
  V_11/1 -> Mux/1
  Demux2/4 -> T_24/1
  Demux2/3 -> T_23/1
  Demux2/2 -> T_22/1
  Demux2/1 -> T_21/1
  Demux1/7 -> P_24/1
  V_22/1 -> Mux/5
  Demux2/7 -> T_27/1
  Demux/5 -> Demux4/1
  Demux/1 -> Demux1/1
  Demux2/8 -> T_28/1
  Demux4/2 -> C_2/1
  Demux/3 -> Demux2/1
  Demux/4 -> Demux3/1
  Modbus Read/1 -> Demux/1
  Demux2/6 -> T_26/1

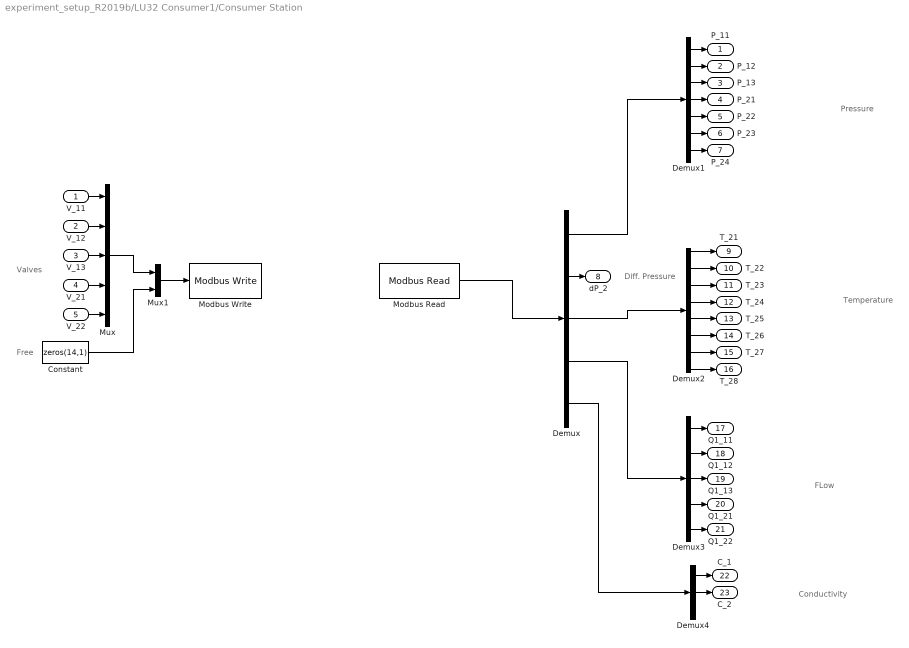
== system experiment_setup_R2019b/LU32 Consumer1/Consumer Station ==
  note: Pressure
  note: Temperature
  note: FLow
  note: Conductivity
  note: Valves
  note: Diff. Pressure
  note: Free
  V_11 : Inport
  V_12 : Inport  Port=2
  V_13 : Inport  Port=3
  V_21 : Inport  Port=4
  V_22 : Inport  Port=5
  Constant : Constant  Value=zeros(14,1)
  Demux : Demux  Outputs=[7 1 8 5 3]
  Demux1 : Demux  Outputs=7
  Demux2 : Demux  Outputs=8
  Demux3 : Demux  Outputs=5
  Demux4 : Demux  Outputs=3
  Modbus Read : modbusMatLib/Modbus Read  registry=0  ipAddress='192.168.100.33'  port=502
  Modbus Write : modbusMatLib/Modbus Write  registry=001  port=502  ipAddress='192.168.100.33'
  Mux : Mux  Inputs=5
  Mux1 : Mux  Inputs=2
  P_11 : Outport  VectorParamsAs1DForOutWhenUnconnected=off
  P_12 : Outport  Port=2  VectorParamsAs1DForOutWhenUnconnected=off
  P_13 : Outport  Port=3  VectorParamsAs1DForOutWhenUnconnected=off
  P_21 : Outport  Port=4  VectorParamsAs1DForOutWhenUnconnected=off
  P_22 : Outport  Port=5  VectorParamsAs1DForOutWhenUnconnected=off
  P_23 : Outport  Port=6  VectorParamsAs1DForOutWhenUnconnected=off
  P_24 : Outport  Port=7  VectorParamsAs1DForOutWhenUnconnected=off
  dP_2 : Outport  Port=8  VectorParamsAs1DForOutWhenUnconnected=off
  T_21 : Outport  Port=9  VectorParamsAs1DForOutWhenUnconnected=off
  T_22 : Outport  Port=10  VectorParamsAs1DForOutWhenUnconnected=off
  T_23 : Outport  Port=11  VectorParamsAs1DForOutWhenUnconnected=off
  T_24 : Outport  Port=12  VectorParamsAs1DForOutWhenUnconnected=off
  T_25 : Outport  Port=13  VectorParamsAs1DForOutWhenUnconnected=off
  T_26 : Outport  Port=14  VectorParamsAs1DForOutWhenUnconnected=off
  T_27 : Outport  Port=15  VectorParamsAs1DForOutWhenUnconnected=off
  T_28 : Outport  Port=16  VectorParamsAs1DForOutWhenUnconnected=off
  Q1_11 : Outport  Port=17  VectorParamsAs1DForOutWhenUnconnected=off
  Q1_12 : Outport  Port=18  VectorParamsAs1DForOutWhenUnconnected=off
  Q1_13 : Outport  Port=19  VectorParamsAs1DForOutWhenUnconnected=off
  Q1_21 : Outport  Port=20  VectorParamsAs1DForOutWhenUnconnected=off
  Q1_22 : Outport  Port=21  VectorParamsAs1DForOutWhenUnconnected=off
  C_1 : Outport  Port=22  VectorParamsAs1DForOutWhenUnconnected=off
  C_2 : Outport  Port=23  VectorParamsAs1DForOutWhenUnconnected=off
  wires:
  Mux/1 -> Mux1/1
  Mux1/1 -> Modbus Write/1
  Constant/1 -> Mux1/2
  Demux1/5 -> P_22/1
  V_12/1 -> Mux/2
  Demux1/6 -> P_23/1
  Demux1/3 -> P_13/1
  Demux1/4 -> P_21/1
  V_13/1 -> Mux/3
  Demux3/2 -> Q1_12/1
  Demux3/5 -> Q1_22/1
  Demux/2 -> dP_2/1
  Demux3/1 -> Q1_11/1
  Demux1/2 -> P_12/1
  Demux2/5 -> T_25/1
  Demux4/1 -> C_1/1
  V_21/1 -> Mux/4
  Demux3/3 -> Q1_13/1
  Demux1/1 -> P_11/1
  Demux3/4 -> Q1_21/1
  V_11/1 -> Mux/1
  Demux2/4 -> T_24/1
  Demux2/3 -> T_23/1
  Demux2/2 -> T_22/1
  Demux2/1 -> T_21/1
  Demux1/7 -> P_24/1
  V_22/1 -> Mux/5
  Demux2/7 -> T_27/1
  Demux/5 -> Demux4/1
  Demux/1 -> Demux1/1
  Demux2/8 -> T_28/1
  Demux4/2 -> C_2/1
  Demux/3 -> Demux2/1
  Demux/4 -> Demux3/1
  Modbus Read/1 -> Demux/1
  Demux2/6 -> T_26/1

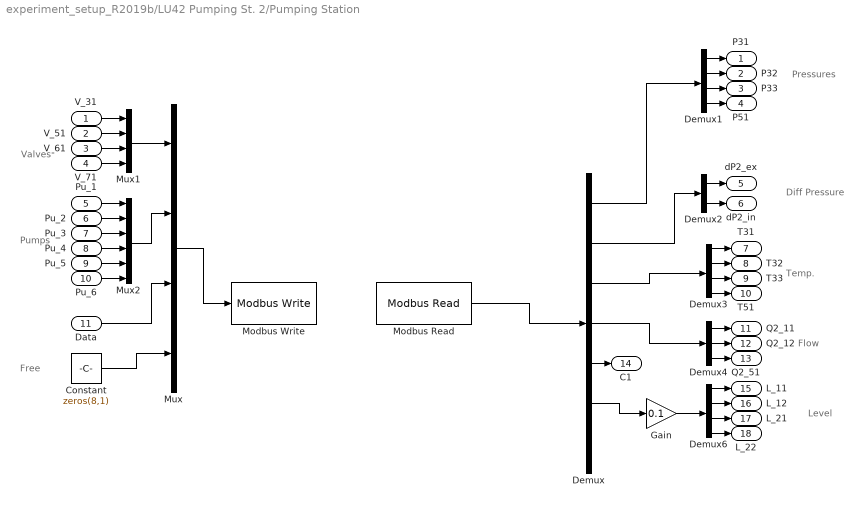
== system experiment_setup_R2019b/LU42 Pumping St. 2/Pumping Station ==
  note: Free
  note: Pumps
  note: Valves
  note: Flow
  note: Temp.
  note: Diff Pressure
  note: Pressures
  note: Level
  V_31 : Inport
  V_51 : Inport  Port=2
  V_61 : Inport  Port=3
  V_71 : Inport  Port=4
  Pu_1 : Inport  Port=5
  Pu_2 : Inport  Port=6
  Pu_3 : Inport  Port=7
  Pu_4 : Inport  Port=8
  Pu_5 : Inport  Port=9
  Pu_6 : Inport  Port=10
  Data : Inport  Port=11
  Constant : Constant  Value=zeros(8,1)
  Demux : Demux  Outputs=[4 2 4 3 1 4 6]
  Demux1 : Demux
  Demux2 : Demux  Outputs=2
  Demux3 : Demux
  Demux4 : Demux  Outputs=3
  Demux6 : Demux
  Gain : Gain  Gain=0.1
  Modbus Read : modbusMatLib/Modbus Read  registry=0  ipAddress='192.168.100.42'  port=502
  Modbus Write : modbusMatLib/Modbus Write  registry=001  port=502  ipAddress='192.168.100.42'
  Mux : Mux
  Mux1 : Mux
  Mux2 : Mux  Inputs=6
  P31 : Outport  VectorParamsAs1DForOutWhenUnconnected=off
  P32 : Outport  Port=2  VectorParamsAs1DForOutWhenUnconnected=off
  P33 : Outport  Port=3  VectorParamsAs1DForOutWhenUnconnected=off
  P51 : Outport  Port=4  VectorParamsAs1DForOutWhenUnconnected=off
  dP2_ex : Outport  Port=5  VectorParamsAs1DForOutWhenUnconnected=off
  dP2_in : Outport  Port=6  VectorParamsAs1DForOutWhenUnconnected=off
  T31 : Outport  Port=7  VectorParamsAs1DForOutWhenUnconnected=off
  T32 : Outport  Port=8  VectorParamsAs1DForOutWhenUnconnected=off
  T33 : Outport  Port=9  VectorParamsAs1DForOutWhenUnconnected=off
  T51 : Outport  Port=10  VectorParamsAs1DForOutWhenUnconnected=off
  Q2_11 : Outport  Port=11  VectorParamsAs1DForOutWhenUnconnected=off
  Q2_12 : Outport  Port=12  VectorParamsAs1DForOutWhenUnconnected=off
  Q2_51 : Outport  Port=13  VectorParamsAs1DForOutWhenUnconnected=off
  C1 : Outport  Port=14  VectorParamsAs1DForOutWhenUnconnected=off
  L_11 : Outport  Port=15  VectorParamsAs1DForOutWhenUnconnected=off
  L_12 : Outport  Port=16  VectorParamsAs1DForOutWhenUnconnected=off
  L_21 : Outport  Port=17  VectorParamsAs1DForOutWhenUnconnected=off
  L_22 : Outport  Port=18  VectorParamsAs1DForOutWhenUnconnected=off
  wires:
  Demux4/1 -> Q2_11/1
  Demux/2 -> Demux2/1
  Demux/4 -> Demux4/1
  Demux2/1 -> dP2_ex/1
  Demux/3 -> Demux3/1
  Demux/1 -> Demux1/1
  Demux3/4 -> T51/1
  Demux1/4 -> P51/1
  Demux3/2 -> T32/1
  Modbus Read/1 -> Demux/1
  Demux6/1 -> L_11/1
  Demux6/2 -> L_12/1
  Demux4/3 -> Q2_51/1
  Demux4/2 -> Q2_12/1
  Demux6/3 -> L_21/1
  Demux6/4 -> L_22/1
  Demux3/3 -> T33/1
  Demux1/1 -> P31/1
  Demux1/2 -> P32/1
  Demux/5 -> C1/1
  Demux1/3 -> P33/1
  Demux2/2 -> dP2_in/1
  Demux3/1 -> T31/1
  Mux/1 -> Modbus Write/1
  Mux1/1 -> Mux/1
  V_31/1 -> Mux1/1
  V_51/1 -> Mux1/2
  V_61/1 -> Mux1/3
  V_71/1 -> Mux1/4
  Pu_4/1 -> Mux2/4
  Pu_3/1 -> Mux2/3
  Pu_1/1 -> Mux2/1
  Pu_2/1 -> Mux2/2
  Mux2/1 -> Mux/2
  Pu_5/1 -> Mux2/5
  Pu_6/1 -> Mux2/6
  Data/1 -> Mux/3
  Constant/1 -> Mux/4
  Gain/1 -> Demux6/1
  Demux/6 -> Gain/1

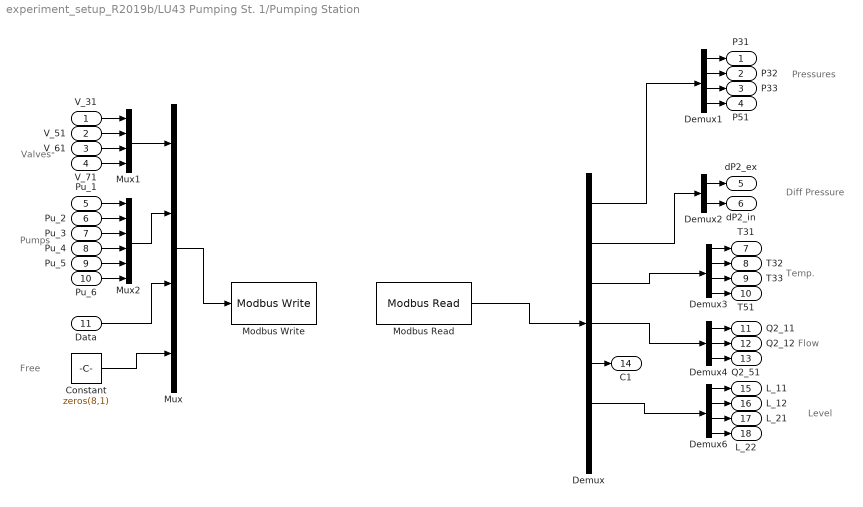
== system experiment_setup_R2019b/LU43 Pumping St. 1/Pumping Station ==
  note: Free
  note: Pumps
  note: Valves
  note: Flow
  note: Temp.
  note: Diff Pressure
  note: Pressures
  note: Level
  V_31 : Inport
  V_51 : Inport  Port=2
  V_61 : Inport  Port=3
  V_71 : Inport  Port=4
  Pu_1 : Inport  Port=5
  Pu_2 : Inport  Port=6
  Pu_3 : Inport  Port=7
  Pu_4 : Inport  Port=8
  Pu_5 : Inport  Port=9
  Pu_6 : Inport  Port=10
  Data : Inport  Port=11
  Constant : Constant  Value=zeros(8,1)
  Demux : Demux  Outputs=[4 2 4 3 1 4 6]
  Demux1 : Demux
  Demux2 : Demux  Outputs=2
  Demux3 : Demux
  Demux4 : Demux  Outputs=3
  Demux6 : Demux
  Modbus Read : modbusMatLib/Modbus Read  registry=0  ipAddress='192.168.100.43'  port=502
  Modbus Write : modbusMatLib/Modbus Write  registry=001  port=502  ipAddress='192.168.100.43'
  Mux : Mux
  Mux1 : Mux
  Mux2 : Mux  Inputs=6
  P31 : Outport  VectorParamsAs1DForOutWhenUnconnected=off
  P32 : Outport  Port=2  VectorParamsAs1DForOutWhenUnconnected=off
  P33 : Outport  Port=3  VectorParamsAs1DForOutWhenUnconnected=off
  P51 : Outport  Port=4  VectorParamsAs1DForOutWhenUnconnected=off
  dP2_ex : Outport  Port=5  VectorParamsAs1DForOutWhenUnconnected=off
  dP2_in : Outport  Port=6  VectorParamsAs1DForOutWhenUnconnected=off
  T31 : Outport  Port=7  VectorParamsAs1DForOutWhenUnconnected=off
  T32 : Outport  Port=8  VectorParamsAs1DForOutWhenUnconnected=off
  T33 : Outport  Port=9  VectorParamsAs1DForOutWhenUnconnected=off
  T51 : Outport  Port=10  VectorParamsAs1DForOutWhenUnconnected=off
  Q2_11 : Outport  Port=11  VectorParamsAs1DForOutWhenUnconnected=off
  Q2_12 : Outport  Port=12  VectorParamsAs1DForOutWhenUnconnected=off
  Q2_51 : Outport  Port=13  VectorParamsAs1DForOutWhenUnconnected=off
  C1 : Outport  Port=14  VectorParamsAs1DForOutWhenUnconnected=off
  L_11 : Outport  Port=15  VectorParamsAs1DForOutWhenUnconnected=off
  L_12 : Outport  Port=16  VectorParamsAs1DForOutWhenUnconnected=off
  L_21 : Outport  Port=17  VectorParamsAs1DForOutWhenUnconnected=off
  L_22 : Outport  Port=18  VectorParamsAs1DForOutWhenUnconnected=off
  wires:
  Demux4/1 -> Q2_11/1
  Demux/2 -> Demux2/1
  Demux/4 -> Demux4/1
  Demux2/1 -> dP2_ex/1
  Demux/3 -> Demux3/1
  Demux/6 -> Demux6/1
  Demux/1 -> Demux1/1
  Demux3/4 -> T51/1
  Demux1/4 -> P51/1
  Demux3/2 -> T32/1
  Modbus Read/1 -> Demux/1
  Demux6/1 -> L_11/1
  Demux6/2 -> L_12/1
  Demux4/3 -> Q2_51/1
  Demux4/2 -> Q2_12/1
  Demux6/3 -> L_21/1
  Demux6/4 -> L_22/1
  Demux3/3 -> T33/1
  Demux1/1 -> P31/1
  Demux1/2 -> P32/1
  Demux/5 -> C1/1
  Demux1/3 -> P33/1
  Demux2/2 -> dP2_in/1
  Demux3/1 -> T31/1
  Mux/1 -> Modbus Write/1
  Mux1/1 -> Mux/1
  V_31/1 -> Mux1/1
  V_51/1 -> Mux1/2
  V_61/1 -> Mux1/3
  V_71/1 -> Mux1/4
  Pu_4/1 -> Mux2/4
  Pu_3/1 -> Mux2/3
  Pu_1/1 -> Mux2/1
  Pu_2/1 -> Mux2/2
  Mux2/1 -> Mux/2
  Pu_5/1 -> Mux2/5
  Pu_6/1 -> Mux2/6
  Data/1 -> Mux/3
  Constant/1 -> Mux/4

== matlab function experiment_setup_R2019b/MATLAB Function ==
  data: dp_tank2 input; pump2_setting output; old_setting input
function pump2_setting = controller(dp_tank2, old_setting)

    if dp_tank2<200                       
        pump2_setting=0;                               
    elseif dp_tank2 > 600
        pump2_setting = 12;
    elseif dp_tank2 > 400
        %pump2_setting = 4;
        pump2_setting = 10;
    else
        pump2_setting = old_setting;
    end
end

== matlab function experiment_setup_R2019b/MATLAB Function1 ==
  settings: updateMethod=DISCRETE
  data: dp_tank1 input; pump1_setting output
function pump1_setting = controller(dp_tank1)
    if dp_tank1<160                       
        pump1_setting=0;
    else
%         pump1_setting = round(rand)*4;
        pump1_setting = 8;
    end
end

== matlab function experiment_setup_R2019b/MATLAB Function3 ==
  settings: updateMethod=DISCRETE
  data: dist_tank_mm input; dist_aux_setting output
function dist_aux_setting = controller(dist_tank_mm)
    if dist_tank_mm<160                       
        dist_aux_setting=0;
    else
        dist_aux_setting = 5+5*rand;
        %pump1_setting = 5;
    end
end

== matlab function experiment_setup_R2019b/MATLAB Function4 ==
  data: buffer_tank_level input; open_buffer_tank output; disturbance_tank_level input; old_output input
function open_buffer_tank = buffers_control(buffer_tank_level, disturbance_tank_level, old_output)

if buffer_tank_level > 600
    open_buffer_tank = 0;
elseif disturbance_tank_level > 600
    open_buffer_tank = 1;
elseif buffer_tank_level < 250
    open_buffer_tank = 1;
elseif disturbance_tank_level < 250
    open_buffer_tank = 0;
else
    open_buffer_tank = old_output;
end
end

== matlab function experiment_setup_R2019b/MATLAB Function2 ==
  data: dp_tank1 input; pump_aux_setting output; old_setting input
function pump_aux_setting = controller(dp_tank1,old_setting)

    if dp_tank1<300                       
        pump_aux_setting = 8;                               
    elseif  dp_tank1 > 550
        pump_aux_setting = 0;
    else
        pump_aux_setting = old_setting;
    end
end
